simulink model "RobotX_Simul_2015a"  (R2015a)
settings: Solver=ode45  StartTime=0.0  StopTime=inf  RelTol=1e-3
libraries: vrlib x4, simulink x3, RobotX_Lib x1
settings Model: CovModelRefEnable=off  Creator=jorgemartins  LastModifiedBy=jorgemartins
settings DataIOCC: SaveFormat=Dataset
settings HardwareCC: ProdBitPerPointer=64  ProdLargestAtomicFloat=Float  ProdIntDivRoundTo=Zero  ProdEndianess=LittleEndian  ProdHWDeviceType=Specified
settings GRTTargetCC: GeneratePreprocessorConditionals=Use local settings

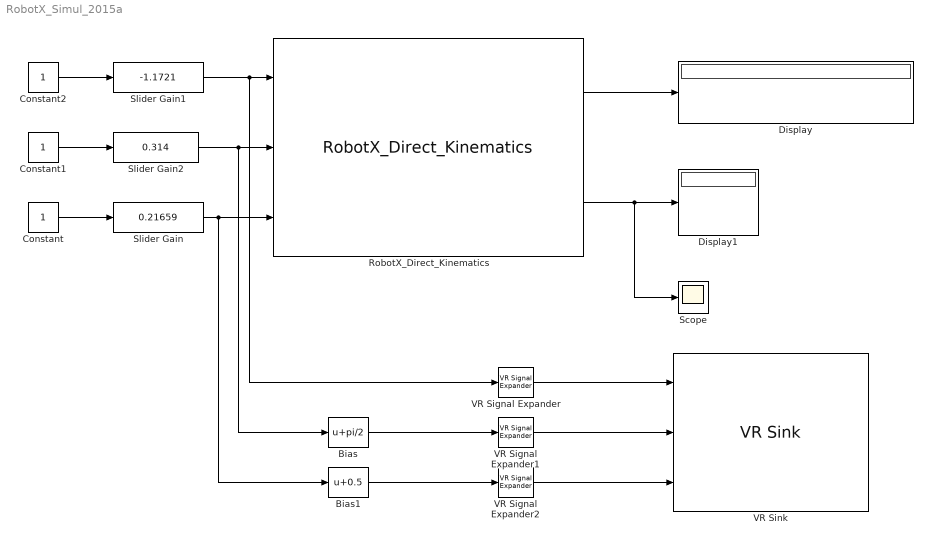
== system RobotX_Simul_2015a ==
  Bias : Bias  Bias=pi/2
  Bias1 : Bias  Bias=0.5
  Constant : Constant
  Constant1 : Constant
  Constant2 : Constant
  Display : Display
  Display1 : Display
  RobotX_Direct_Kinematics : RobotX_Lib/RobotX_Direct_Kinematics
  Scope : Scope
      settings: TimeRange=auto  MaxDataPoints=5000  SaveToWorkspace=off  SaveName=ScopeData  YMin=-0.63361  YMax=0.84472  SampleTime=-1
  Slider Gain : simulink/Math Operations/Slider Gain  low=-1  gain=0.21659  high=1
  Slider Gain1 : simulink/Math Operations/Slider Gain  low=-3.14  gain=-1.1721  high=3.14
  Slider Gain2 : simulink/Math Operations/Slider Gain  low=-3.14  gain=0.314  high=3.14
  VR Signal Expander : vrlib/VR Signal Expander  outwidth=4  outidx=[4]
  VR Signal Expander1 : vrlib/VR Signal Expander  outwidth=4  outidx=[4]
  VR Signal Expander2 : vrlib/VR Signal Expander  outwidth=3  outidx=[3]
  VR Sink : vrlib/VR Sink  InstantiateOnLoad=on  SampleTime=-1  ViewEnable=on  RemoteChange=off  RemoteView=off  FieldsWritten=Jt1_DH_dv.rotation.4.1.1.double#Jt2_DH_dv.rotation.4.1.1.double#Jt3_DH_dv.translation.3.1.1.double  WorldFileName=vrrobot.wrl  WorldDescription=D-H Reference Frames for Virtual Reality Robot  AutoView=on  VideoDimensions=[]  AllowVariableSize=off  FigureProperties="{'Position', 'Name', 'Viewpoint', 'CameraBound', 'CameraDirection', 'CameraPosition', 'CameraUpVector', 'ZoomFactor', 'Antialiasing', 'Headlight', 'Lighting', 'NavPanel', 'Sound', 'StatusBar', 'Stereo3D', 'Stereo3DCameraOffset', 'Stereo3DHIT', 'ToolBar', 'Textures', 'Transparency', 'Triad', 'Wireframe', 'NavZones', 'NavMode', 'NavSpeed', 'CaptureFileFormat', 'CaptureFileName', 'Record2DCompressMethod', 'Record2DCompressQuality', 'Record2D', 'Record2DFileName', 'Record2DFPS'; [5.0000000000000000e+00   9.5000000000000000e+01   5.7600000000000000e+02   3.8000000000000000e+02], 'D-H Reference Frames for Virtual Reality Robot', 'View 1', 'on', [-8.0791469061357979e-01   2.0126392539898955e-01  -5.5386522279675776e-01], [2.7692368285477924e+00  -9.3485769358792326e-01   2.4254062784801578e-01], [1.0652040279345899e-01   9.7426477316967686e-01   1.9864932808670713e-01], [1.0000000000000000e+00], 'on', 'on', 'on', 'halfbar', 'on', 'on', 'off', [1.0000000149011612e-01], [0.0000000000000000e+00], 'on', 'on', 'on', 'none', 'off', 'off', 'examine', 'normal', 'tif', '%f_anim_%n.tif', 'auto', [7.5000000000000000e+01], 'off', '%f_anim_%n.avi', 'auto'}"
  wires:
  RobotX_Direct_Kinematics/1 -> Display/1
  RobotX_Direct_Kinematics/2 -> Scope/1, Display1/1
  Constant/1 -> Slider Gain/1
  Slider Gain/1 -> Bias1/1, RobotX_Direct_Kinematics/3
  Constant2/1 -> Slider Gain1/1
  Slider Gain1/1 -> VR Signal Expander/1, RobotX_Direct_Kinematics/1
  Constant1/1 -> Slider Gain2/1
  Slider Gain2/1 -> Bias/1, RobotX_Direct_Kinematics/2
  VR Signal Expander/1 -> VR Sink/1
  VR Signal Expander1/1 -> VR Sink/2
  VR Signal Expander2/1 -> VR Sink/3
  Bias/1 -> VR Signal Expander1/1
  Bias1/1 -> VR Signal Expander2/1
